simulink model "mrsMultiRobotAvoidance"  (R2024a)
settings: Solver=FixedStepAuto  StartTime=0.0  StopTime=inf  FixedStep=sampleTime  RelTol=1e-3
PreLoadFcn:
  | % Simulation parameters
  | load exampleMap
  | sampleTime = 0.05;
  | 
  | % Robot parameters
  | wheelRadius = 0.025;
  | robotRadius = 0.35;
  | 
  | % Lidar parameters
  | sensorOffset = [0,0];
  | scanAngles = linspace(-pi/2,pi/2,9)';
  | maxRange = 5;
undefined symbols (not defined in the file): detect_array, objDetectorAngle, objDetectorFOV, objDetectorOffset, objDetectorRange
libraries: mobileRoboticsLib x10
settings Model: Creator=scastro  LastModifiedBy=niyu2
settings SolverCC: AlgebraicLoopSolver=TrustRegion
settings DataIOCC: ReturnWorkspaceOutputs=off
settings DebuggingCC: UnconnectedInputMsg=warning  UnconnectedOutputMsg=warning  UnconnectedLineMsg=warning  PregeneratedLibrarySubsystemCodeDiagnostic=none  ArithmeticOperatorsInVariantConditions=warning
settings ModelReferenceCC: EnableRefExpFcnMdlSchedulingChecks=on
settings SFSimCC: SimUseLocalCustomCode=off  CustomCodeUndefinedFunction=UseInterfaceOnly
settings RTWCC: RTWUseLocalCustomCode=off  GPUComputeCapability=3.5

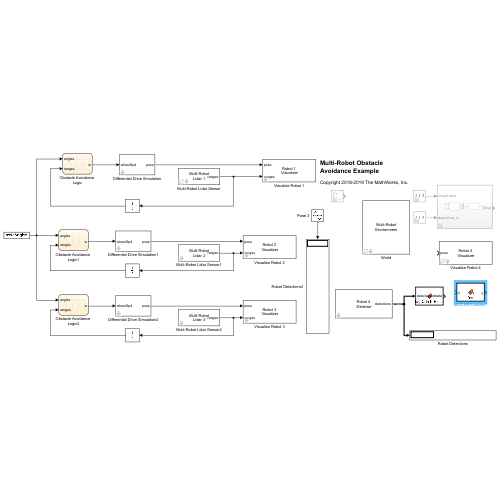
[thumbnail: Simulink's stored preview of the top-level diagram]
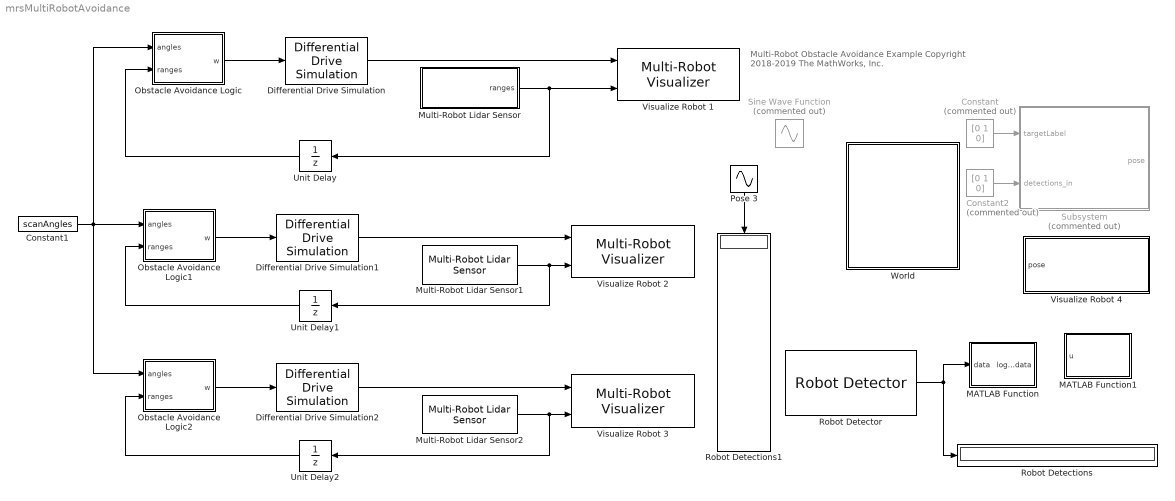
== system mrsMultiRobotAvoidance ==
  note: Multi-Robot Obstacle
      | Avoidance Example
      |
      | Copyright 2018-2019 The MathWorks, Inc.
  Constant : Constant  Commented=on  Value=[0 1 0]
  Constant1 : Constant  Value=scanAngles
  Constant2 : Constant  Commented=on  Value=[0 1 0]
  Differential Drive Simulation : mobileRoboticsLib/Kinematic Models/Differential Drive/Differential Drive Simulation  wheelRadius=wheelRadius  wheelBase=robotRadius  initX=4  initY=4  initAngle=0  Ts=sampleTime
      settings: SourceProductName=Mobile Robotics Simulation Toolbox
  Differential Drive Simulation1 : mobileRoboticsLib/Kinematic Models/Differential Drive/Differential Drive Simulation  wheelRadius=wheelRadius  wheelBase=robotRadius  initX=8  initY=8  initAngle=pi/2  Ts=sampleTime
      settings: SourceProductName=Mobile Robotics Simulation Toolbox
  Differential Drive Simulation2 : mobileRoboticsLib/Kinematic Models/Differential Drive/Differential Drive Simulation  wheelRadius=wheelRadius  wheelBase=robotRadius  initX=7.5  initY=3  initAngle=-pi/4  Ts=sampleTime
      settings: SourceProductName=Mobile Robotics Simulation Toolbox
  MATLAB Function : MATLAB Function  TreatAsAtomicUnit=on
  MATLAB Function1 : MATLAB Function  TreatAsAtomicUnit=on
  Multi-Robot Lidar Sensor : Subsystem  AncestorBlock=mobileRoboticsLib/Environments/Multi-Robot Lidar Sensor  mask(Multi-Robot Lidar Sensor){robotIdx=1, mapName=map, sensorOffset=sensorOffset, scanAngles=scanAngles, maxRange=maxRange}
      mask prompts: robotIdx "Robot Index"; mapName "Map Name"; sensorOffset "Sensor offset (x,y) [m]"; scanAngles "Scan angles [rad]"; maxRange "Maximum Range [m]"
      mask help: 2D lidar sensor simulation for multi-robot environment.
      mask init:
      | % Find number of robots 
      | mrEnvBlks = find_system(bdroot,'FollowLinks','on','LookUnderMasks','on','MaskType','Multi-Robot Environment');
      | mrEnvBlk = mrEnvBlks{1};
      | if isempty(mrEnvBlk)
      |     error('No Multi-Robot Environment found in model.')
      | end
      | numRobots = evalin('base',get_param(mrEnvBlk,'numRobots'));
      | 
      | % Configure pose tags
      | poseSub = [gcb '/Poses'];
      | poseBlocks = find_system(poseSub,'FollowLinks','on','LookUnderMasks','on','BlockType','From');
      | for idx = 1:numel(poseBlocks)
      |     lh = get_param(poseBlocks{idx},'LineHandles');
      |     delete_line(lh.Outport);
      | end
      | delete_block(poseBlocks);
      | vecBlock = [poseSub '/Vector Concatenate'];
      | set_param(vecBlock,'NumInputs',num2str(numRobots));
      | for idx = 1:numRobots
      |     blkName = [poseSub '/From' num2str(idx)];
      |     blkPos = [0 30 200 50] + (idx-1)*[0 30 0 30];
      |     add_block('simulink/Signal Routing/From',blkName);
      |     set_param(blkName,'GotoTag',['slMultiRobotEnv_Pose_' num2str(idx)]);
      |     set_param(blkName,'Position',blkPos);
      |     add_line(poseSub,['From' num2str(idx) '/1'],['Vector Concatenate/' num2str(idx)]);
      | end
      | 
      | % Configure visual tags
      | visualSub = [gcb '/Visuals'];
      | visualBlocks = find_system(visualSub,'FollowLinks','on','LookUnderMasks','on','BlockType','From');
      | for idx = 1:numel(visualBlocks)
      |     lh = get_param(visualBlocks{idx},'LineHandles');
      |     delete_line(lh.Outport);
      | end
      | delete_block(visualBlocks);
      | vecBlock = [visualSub '/Vector Concatenate'];
      | set_param(vecBlock,'NumInputs',num2str(numRobots));
      | for idx = 1:numRobots
      |     blkName = [visualSub '/From' num2str(idx)];
      |     blkPos = [0 30 200 50] + (idx-1)*[0 30 0 30];
      |     add_block('simulink/Signal Routing/From',blkName);
      |     set_param(blkName,'GotoTag',['slMultiRobotEnv_Visuals_' num2str(idx)]);
      |     set_param(blkName,'Position',blkPos);
      |     add_line(visualSub,['From' num2str(idx) '/1'],['Vector Concatenate/' num2str(idx)]);
      | end
      mask Help: web('matlab: edit mrsDocLidarSensor')
      mask Callback mapName:
      | % Update the map in the Robot Detector system object inside the mask
      | mapName = get_param(gcb,'mapName');
      | blkName = [gcb '/Multi-Robot Lidar Sensor'];
      | set_param(blkName,'mapName',mapName);
      mask Display:
      | idx = get_param(gcb,'robotIdx');
      | fprintf(['Multi Robot\nLidar ' idx])
  Multi-Robot Lidar Sensor1 : mobileRoboticsLib/Environments/Multi-Robot Lidar Sensor  robotIdx=2  mapName=map  sensorOffset=sensorOffset  scanAngles=scanAngles  maxRange=maxRange
      settings: SourceProductName=Mobile Robotics Simulation Toolbox
  Multi-Robot Lidar Sensor2 : mobileRoboticsLib/Environments/Multi-Robot Lidar Sensor  robotIdx=3  mapName=map  sensorOffset=sensorOffset  scanAngles=scanAngles  maxRange=maxRange
      settings: SourceProductName=Mobile Robotics Simulation Toolbox
  Obstacle Avoidance Logic : Stateflow chart  TreatAsAtomicUnit=on
  Obstacle Avoidance Logic1 : Stateflow chart  TreatAsAtomicUnit=on
  Obstacle Avoidance Logic2 : Stateflow chart  TreatAsAtomicUnit=on
  Pose 3 : Sin  SineType=Sample based  Amplitude=[-2;0.5;pi/2]  Bias=[7.75;3;0]  Phase=[-pi/4;0;pi/3]  Samples=160  SampleTime=sampleTime  Offset=[0;50;25]
  Robot Detections : Display
  Robot Detections1 : Display
  Robot Detector : mobileRoboticsLib/Environments/Robot Detector  mapName=map  robotIdx=4  sensorOffset=[0,0]  sensorAngle=0  sensorFOV=pi/3  maxRange=10  maxDetections=1  sampleTime=-1
      settings: SourceProductName=Mobile Robotics Simulation Toolbox
  Sine Wave Function : Sin  Commented=on  SineType=Sample based  Amplitude=[detect_array(1);detect_array(2);detect_array(3)]  Bias=[7.75;3;0]  Samples=160  SampleTime=0.05  Offset=[0;50;25]
  Subsystem : Subsystem  Commented=on
  Unit Delay : UnitDelay  SampleTime=-1  HasFrameUpgradeWarning=on
  Unit Delay1 : UnitDelay  SampleTime=-1  HasFrameUpgradeWarning=on
  Unit Delay2 : UnitDelay  SampleTime=-1  HasFrameUpgradeWarning=on
  Visualize Robot 1 : mobileRoboticsLib/Environments/Multi-Robot Visualizer  idx=1  radius=robotRadius  robotColor=[0 1 0]  showTraj=off  hasLidar=on  sensorOffset=sensorOffset  scanAngles=scanAngles  maxNumScans=0  hasObjDetector=off  objDetectorOffset=[0,0]  objDetectorAngle=0  objDetectorFOV=pi/2  objDetectorMaxRange=5  hasRobotDetector=off  robotDetectorOffset=[0,0]  robotDetectorAngle=0  robotDetectorFOV=pi/3  robotDetectorMaxRange=5  robotDetectorNumDetections=0
      settings: SourceProductName=Mobile Robotics Simulation Toolbox
  Visualize Robot 2 : mobileRoboticsLib/Environments/Multi-Robot Visualizer  idx=2  radius=robotRadius  robotColor=[0 0 1]  showTraj=on  hasLidar=on  sensorOffset=sensorOffset  scanAngles=scanAngles  maxNumScans=0  hasObjDetector=off  objDetectorOffset=[0 0]  objDetectorAngle=0  objDetectorFOV=pi/2  objDetectorMaxRange=5  hasRobotDetector=off  robotDetectorOffset=[0,0]  robotDetectorAngle=0  robotDetectorFOV=pi/3  robotDetectorMaxRange=5  robotDetectorNumDetections=0
      settings: SourceProductName=Mobile Robotics Simulation Toolbox
  Visualize Robot 3 : mobileRoboticsLib/Environments/Multi-Robot Visualizer  idx=3  radius=robotRadius  robotColor=[0 0 1]  showTraj=off  hasLidar=on  sensorOffset=sensorOffset  scanAngles=scanAngles  maxNumScans=0  hasObjDetector=off  objDetectorOffset=[0 0]  objDetectorAngle=0  objDetectorFOV=pi/2  objDetectorMaxRange=5  hasRobotDetector=off  robotDetectorOffset=[0,0]  robotDetectorAngle=0  robotDetectorFOV=pi/3  robotDetectorMaxRange=5  robotDetectorNumDetections=0
      settings: SourceProductName=Mobile Robotics Simulation Toolbox
  Visualize Robot 4 : Subsystem  AncestorBlock=mobileRoboticsLib/Environments/Multi-Robot Visualizer  mask(Multi-Robot Visualizer){idx=4, radius=0.25, robotColor=[0 0 1], showTraj=on, hasLidar=off, sensorOffset=sensorOffset, scanAngles=scanAngles, maxNumScans=0, hasObjDetector=off, objDetectorOffset=objDetectorOffset, objDetectorAngle=objDetectorAngle, objDetectorFOV=objDetectorFOV, objDetectorMaxRange=objDetectorRange, hasRobotDetector=on, robotDetectorOffset=[0,0], robotDetectorAngle=0, robotDetectorFOV=pi/3, robotDetectorMaxRange=10, robotDetectorNumDetections=0}
      mask prompts: idx "Robot Index"; radius "Robot Radius [m]"; robotColor "Robot Color"; showTraj "Show Trajectory"; hasLidar "Accept Lidar"; sensorOffset "Lidar sensor offset (x,y) [m]"; scanAngles "Scan angles [rad]"; maxNumScans "Maximum number of scans"; hasObjDetector "Accept Object Detector"; objDetectorOffset "Object detector offset (x,y) [m]"; objDetectorAngle "Object detector angle [rad]"; objDetectorFOV "Object detector field of view [rad]"; objDetectorMaxRange "Object detector maximum range [m]"; hasRobotDetector "Accept Robot Detector"; robotDetectorOffset "Robot detector offset (x,y) [m]"; robotDetectorAngle "Robot detector angle [rad]"; robotDetectorFOV "Robot detector field of view [rad]"; robotDetectorMaxRange "Robot detector maximum range [m]"; robotDetectorNumDetections "Maximum number of detections"
      mask help:
      | Supply the pose and (optionally) lidar ranges for a single robot in a multi-robot setup.
      |
      | These blocks require a "Multi-Robot Environment" block to exist in the model.
      mask init:
      | % Configure ranges port
      | if ~hasLidar & ~isempty(find_system(gcb,'FollowLinks','on','LookUnderMasks','on','BlockType','Inport','Name','ranges'))
      |     replace_block(gcb,'FollowLinks','on','Name','ranges','built-in/Ground','noprompt');
      | elseif hasLidar & isempty(find_system(gcb,'FollowLinks','on','LookUnderMasks','on','BlockType','Inport','Name','ranges'))
      |     replace_block(gcb,'FollowLinks','on','Name','ranges','built-in/Inport','noprompt');  
      | end
      | 
      | % Set up the Goto tag numbers
      | set_param([gcb '/Goto_Visuals'],'GotoTag',['slMultiRobotEnv_Visuals_' num2str(idx)]);
      | set_param([gcb '/Goto_Pose'],'GotoTag',['slMultiRobotEnv_Pose_' num2str(idx)]);
      | set_param([gcb '/Goto_Ranges'],'GotoTag',['slMultiRobotEnv_Ranges_' num2str(idx)]);
      | set_param([gcb '/Goto_ObjDetector'],'GotoTag',['slMultiRobotEnv_ObjDet_' num2str(idx)]);
      | set_param([gcb '/Goto_RobotDetector'],'GotoTag',['slMultiRobotEnv_RobotDet_' num2str(idx)]);
      | 
      | % Get the maximum number of scans
      | maxNumScans = internal.getMaxNumScans;
      | 
      | % Initialize range sensor bus
      | internal.createRangeSensorBus;
      mask Help: web('matlab: edit mrsDocMultiRobotEnv')
      mask Callback hasLidar:
      | mask = Simulink.Mask.get(gcb);
      | hasLidar = get_param(gcb,'hasLidar');
      | 
      | % Enable and disable parameters
      | indices = [find(strcmp({mask.Parameters.Name},'sensorOffset'));
      |            find(strcmp({mask.Parameters.Name},'scanAngles'))];
      | 
      | for idx = 1:numel(indices)
      |     mask.Parameters(indices(idx)).Visible = hasLidar;
      | end
      mask Callback hasObjDetector:
      | mask = Simulink.Mask.get(gcb);
      | hasObjDetector = get_param(gcb,'hasObjDetector');
      | 
      | indices = [find(strcmp({mask.Parameters.Name},'objDetectorOffset'));
      |            find(strcmp({mask.Parameters.Name},'objDetectorAngle'));
      |            find(strcmp({mask.Parameters.Name},'objDetectorFOV'));
      |            find(strcmp({mask.Parameters.Name},'objDetectorMaxRange'))];
      | 
      | for idx = 1:numel(indices)
      |     mask.Parameters(indices(idx)).Visible = hasObjDetector;
      | end
      mask Callback hasRobotDetector:
      | mask = Simulink.Mask.get(gcb);
      | hasObjDetector = get_param(gcb,'hasRobotDetector');
      | 
      | indices = [find(strcmp({mask.Parameters.Name},'robotDetectorOffset'));
      |            find(strcmp({mask.Parameters.Name},'robotDetectorAngle'));
      |            find(strcmp({mask.Parameters.Name},'robotDetectorFOV'));
      |            find(strcmp({mask.Parameters.Name},'robotDetectorMaxRange'))];
      | 
      | for idx = 1:numel(indices)
      |     mask.Parameters(indices(idx)).Visible = hasObjDetector;
      | end
      mask DialogControl Container4 Prompt: Robot
      mask DialogControl Container6 Prompt: Sensors
      mask Display:
      | idx = get_param(gcb,'idx');
      | fprintf(['Robot ' idx '\n Visualizer'])
  World : Subsystem  AncestorBlock=mobileRoboticsLib/Environments/Multi-Robot Environment  InitFcn=clear multiRobotVizWorld;  mask(Multi-Robot Environment){numRobots=4, mapName=map, showWaypoints=off, showObjects=off, objectColors=[1 0 0;0 1 0;0 0 1], objectMarkers='s', showRobotIds=on, plotSensorLines=on}
      mask prompts: numRobots "Number of Robots"; mapName "Map Name"; showWaypoints "Accept Waypoints"; showObjects "Accept Objects"; objectColors "Object Colors"; objectMarkers "Object Markers"; showRobotIds "Show Robot IDs"; plotSensorLines "Plot Sensor Lines"
      mask help:
      | Displays map, waypoint, and object data for a multi-robot simulation.
      |
      | Use "Multi-Robot Visualizer" blocks to display individual robots in this environment.
      mask init:
      | % Configure visual tags
      | visualSub = [gcb '/Visuals'];
      | radiusBlocks = find_system(visualSub,'FollowLinks','on','LookUnderMasks','on','BlockType','From');
      | for idx = 1:numel(radiusBlocks)
      |     lh = get_param(radiusBlocks{idx},'LineHandles');
      |     delete_line(lh.Outport);
      | end
      | delete_block(radiusBlocks);
      | vecBlock = [visualSub '/Vector Concatenate'];
      | set_param(vecBlock,'NumInputs',num2str(numRobots));
      | for idx = 1:numRobots
      |     blkName = [visualSub '/From' num2str(idx)];
      |     blkPos = [0 30 200 50] + (idx-1)*[0 30 0 30];
      |     add_block('simulink/Signal Routing/From',blkName);
      |     set_param(blkName,'GotoTag',['slMultiRobotEnv_Visuals_' num2str(idx)]);
      |     set_param(blkName,'Position',blkPos);
      |     add_line(visualSub,['From' num2str(idx) '/1'],['Vector Concatenate/' num2str(idx)]);
      | end
      | 
      | % Configure pose tags
      | poseSub = [gcb '/Poses'];
      | poseBlocks = find_system(poseSub,'FollowLinks','on','LookUnderMasks','on','BlockType','From');
      | for idx = 1:numel(poseBlocks)
      |     lh = get_param(poseBlocks{idx},'LineHandles');
      |     delete_line(lh.Outport);
      | end
      | delete_block(poseBlocks);
      | vecBlock = [poseSub '/Vector Concatenate'];
      | set_param(vecBlock,'NumInputs',num2str(numRobots));
      | for idx = 1:numRobots
      |     blkName = [poseSub '/From' num2str(idx)];
      |     blkPos = [0 30 200 50] + (idx-1)*[0 30 0 30];
      |     add_block('simulink/Signal Routing/From',blkName);
      |     set_param(blkName,'GotoTag',['slMultiRobotEnv_Pose_' num2str(idx)]);
      |     set_param(blkName,'Position',blkPos);
      |     add_line(poseSub,['From' num2str(idx) '/1'],['Vector Concatenate/' num2str(idx)]);
      | end
      | 
      | % Configure range tags
      | rangeSub = [gcb '/Ranges'];
      | rangeBlocks = find_system(rangeSub,'FollowLinks','on','LookUnderMasks','on','BlockType','From');
      | for idx = 1:numel(rangeBlocks)
      |     lh = get_param(rangeBlocks{idx},'LineHandles');
      |     delete_line(lh.Outport);
      | end
      | delete_block(rangeBlocks);
      | vecBlock = [rangeSub '/Vector Concatenate'];
      | set_param(vecBlock,'NumInputs',num2str(numRobots));
      | for idx = 1:numRobots
      |     blkName = [rangeSub '/From' num2str(idx)];
      |     blkPos = [0 30 200 50] + (idx-1)*[0 30 0 30];
      |     add_block('simulink/Signal Routing/From',blkName);
      |     set_param(blkName,'GotoTag',['slMultiRobotEnv_Ranges_' num2str(idx)]);
      |     set_param(blkName,'Position',blkPos);
      |     add_line(rangeSub,['From' num2str(idx) '/1'],['Vector Concatenate/' num2str(idx)]);
      | end
      | 
      | % Initialize range sensor bus
      | internal.createRangeSensorBus;
      | 
      | % Configure object detector tags
      | objDetSub = [gcb '/ObjectDetectorParams'];
      | objDetBlocks = find_system(objDetSub,'FollowLinks','on','LookUnderMasks','on','BlockType','From');
      | for idx = 1:numel(objDetBlocks)
      |     lh = get_param(objDetBlocks{idx},'LineHandles');
      |     delete_line(lh.Outport);
      | end
      | delete_block(objDetBlocks);
      | vecBlock = [objDetSub '/Vector Concatenate'];
      | set_param(vecBlock,'NumInputs',num2str(numRobots));
      | for idx = 1:numRobots
      |     blkName = [objDetSub '/From' num2str(idx)];
      |     blkPos = [0 30 200 50] + (idx-1)*[0 30 0 30];
      |     add_block('simulink/Signal Routing/From',blkName);
      |     set_param(blkName,'GotoTag',['slMultiRobotEnv_ObjDet_' num2str(idx)]);
      |     set_param(blkName,'Position',blkPos);
      |     add_line(objDetSub,['From' num2str(idx) '/1'],['Vector Concatenate/' num2str(idx)]);
      | end
      | 
      | % Configure robot detector tags
      | robotDetSub = [gcb '/RobotDetectorParams'];
      | robotDetBlocks = find_system(robotDetSub,'FollowLinks','on','LookUnderMasks','on','BlockType','From');
      | for idx = 1:numel(robotDetBlocks)
      |     lh = get_param(robotDetBlocks{idx},'LineHandles');
      |     delete_line(lh.Outport);
      | end
      | delete_block(robotDetBlocks);
      | vecBlock = [robotDetSub '/Vector Concatenate'];
      | set_param(vecBlock,'NumInputs',num2str(numRobots));
      | for idx = 1:numRobots
      |     blkName = [robotDetSub '/From' num2str(idx)];
      |     blkPos = [0 30 200 50] + (idx-1)*[0 30 0 30];
      |     add_block('simulink/Signal Routing/From',blkName);
      |     set_param(blkName,'GotoTag',['slMultiRobotEnv_RobotDet_' num2str(idx)]);
      |     set_param(blkName,'Position',blkPos);
      |     add_line(robotDetSub,['From' num2str(idx) '/1'],['Vector Concatenate/' num2str(idx)]);
      | end
      | 
      | % Configure waypoints port
      | hasWaypointPort = ~isempty(find_system(gcb,'FollowLinks','on','LookUnderMasks','on','BlockType','Inport','Name','waypoints'));
      | if ~showWaypoints & hasWaypointPort
      |     replace_block(gcb,'FollowLinks','on','Name','waypoints','built-in/Ground','noprompt');
      | elseif showWaypoints & ~hasWaypointPort
      |     replace_block(gcb,'FollowLinks','on','Name','waypoints','built-in/Inport','noprompt'); 
      | end
      |  
      | % Configure objects port
      | hasObjectPort = ~isempty(find_system(gcb,'FollowLinks','on','LookUnderMasks','on','BlockType','Inport','Name','objects'));
      | if ~showObjects & hasObjectPort
      |     replace_block(gcb,'FollowLinks','on','Name','objects','built-in/Ground','noprompt');
      | elseif showObjects & ~hasObjectPort
      |     replace_block(gcb,'FollowLinks','on','Name','objects','built-in/Inport','noprompt');  
      | end
      | 
      | % Ensure the waypoints and objects ports are organized correctly
      | if strcmp(get_param([gcb '/waypoints'],'BlockType'),'Inport')
      |     set_param([gcb '/waypoints'],'Port','1');
      | end
      mask Help: web('matlab: edit mrsDocMultiRobotEnv')
      mask Callback showObjects:
      | mask = Simulink.Mask.get(gcb);
      | showObjects = get_param(gcb,'showObjects');
      | 
      | % Enable and disable parameters
      | indices = [find(strcmp({mask.Parameters.Name},'objectColors'));
      |            find(strcmp({mask.Parameters.Name},'objectMarkers'))];
      | 
      | for idx = 1:numel(indices)
      |     mask.Parameters(indices(idx)).Visible = showObjects;
      | end
      mask Display: fprintf('Multi-Robot\nEnvironment')
  wires:
  Differential Drive Simulation/1 -> Visualize Robot 1/1
  Differential Drive Simulation1/1 -> Visualize Robot 2/1
  Obstacle Avoidance Logic/1(w) -> Differential Drive Simulation/1
  Unit Delay/1 -> Obstacle Avoidance Logic/2(ranges)
  Obstacle Avoidance Logic1/1(w) -> Differential Drive Simulation1/1
  Unit Delay1/1 -> Obstacle Avoidance Logic1/2(ranges)
  Unit Delay2/1 -> Obstacle Avoidance Logic2/2(ranges)
  Constant1/1 -> Obstacle Avoidance Logic2/1(angles), Obstacle Avoidance Logic1/1(angles), Obstacle Avoidance Logic/1(angles)
  Multi-Robot Lidar Sensor2/1 -> Visualize Robot 3/2, Unit Delay2/1
  Obstacle Avoidance Logic2/1(w) -> Differential Drive Simulation2/1
  Differential Drive Simulation2/1 -> Visualize Robot 3/1
  Multi-Robot Lidar Sensor/1(ranges) -> Unit Delay/1, Visualize Robot 1/2
  Multi-Robot Lidar Sensor1/1 -> Unit Delay1/1, Visualize Robot 2/2
  Pose 3/1 -> Robot Detections1/1
  Constant/1 -> Subsystem/1(targetLabel)
  Constant2/1 -> Subsystem/2(detections_in)
  Robot Detector/1 -> MATLAB Function/1(data), Robot Detections/1

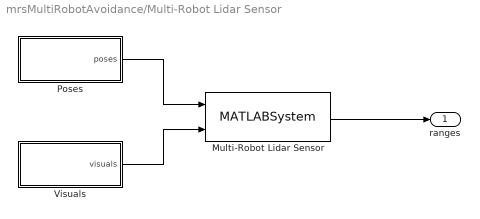
== system mrsMultiRobotAvoidance/Multi-Robot Lidar Sensor ==
  Multi-Robot Lidar Sensor : MATLABSystem  System=MultiRobotLidarSensor  mapName=map  sensorOffset=sensorOffset  scanAngles=scanAngles  maxRange=maxRange  robotIdx=robotIdx  robotRadii=-1
      mask Type: MultiRobotLidarSensor
      mask Display:
      | disp(['Multi-Robot' char(10) 'Lidar 1']);
      | port_label('output',1,'ranges');
  Poses : Subsystem
  Visuals : Subsystem
  ranges : Outport  VectorParamsAs1DForOutWhenUnconnected=off
  wires:
  Visuals/1(visuals) -> Multi-Robot Lidar Sensor/2
  Multi-Robot Lidar Sensor/1 -> ranges/1
  Poses/1(poses) -> Multi-Robot Lidar Sensor/1

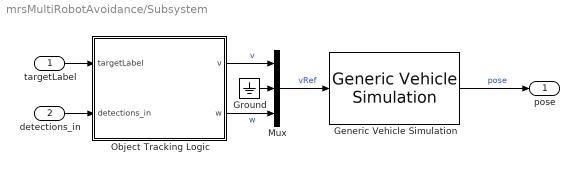
== system mrsMultiRobotAvoidance/Subsystem ==
  targetLabel : Inport
  detections_in : Inport  Port=2
  Generic Vehicle Simulation : mobileRoboticsLib/Utilities/Generic Vehicle Simulation  initX=2  initY=3  initAngle=0  Ts=sampleTime
      settings: SourceProductName=Mobile Robotics Simulation Toolbox
  Ground : Ground
  Mux : Mux  Inputs=3
  Object Tracking Logic : Stateflow chart  TreatAsAtomicUnit=on
  pose : Outport
  wires:
  targetLabel/1 -> Object Tracking Logic/1(targetLabel)
  Mux/1 -> Generic Vehicle Simulation/1  "vRef"
  Object Tracking Logic/2(w) -> Mux/3  "w"
  Object Tracking Logic/1(v) -> Mux/1  "v"
  detections_in/1 -> Object Tracking Logic/2(detections_in)
  Ground/1 -> Mux/2
  Generic Vehicle Simulation/1 -> pose/1  "pose"

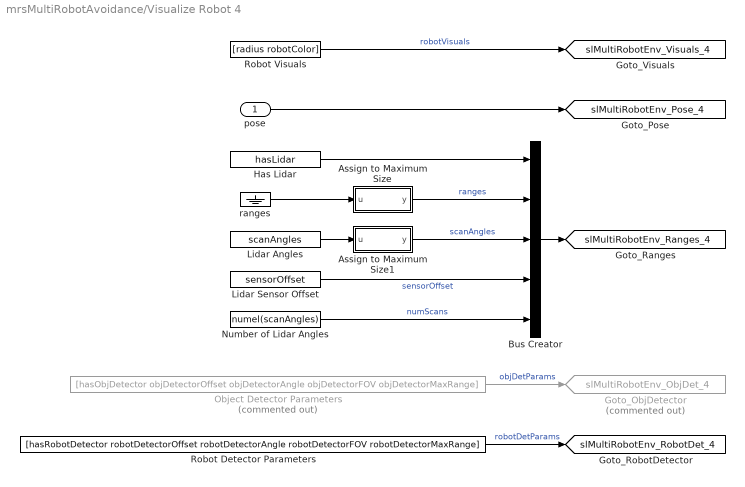
== system mrsMultiRobotAvoidance/Visualize Robot 4 ==
  pose : Inport
  Assign to Maximum Size : MATLAB Function  TreatAsAtomicUnit=on  mask{maxLength=maxNumScans}
      mask prompts: maxLength "Maximum Length"
  Assign to Maximum Size1 : MATLAB Function  TreatAsAtomicUnit=on  mask{maxLength=maxNumScans}
      mask prompts: maxLength "Maximum Length"
  Bus Creator : BusCreator  Inputs=5  OutDataTypeStr=Bus: slbus_MultiRobotRangeSensor  NonVirtualBus=on
      settings: InheritFromInputs=off
  Goto_ObjDetector : Goto  Commented=on  GotoTag=slMultiRobotEnv_ObjDet_4  TagVisibility=global
  Has Lidar : Constant  Value=hasLidar  OutDataTypeStr=boolean
  Lidar Angles : Constant  Value=scanAngles
  Lidar Sensor Offset : Constant  Value=sensorOffset
  Number of Lidar Angles : Constant  Value=numel(scanAngles)
  Object Detector Parameters : Constant  Commented=on  Value=[hasObjDetector objDetectorOffset objDetectorAngle objDetectorFOV objDetectorMaxRange]
  Robot Detector Parameters : Constant  Value=[hasRobotDetector robotDetectorOffset robotDetectorAngle robotDetectorFOV robotDetectorMaxRange]
  Robot Visuals : Constant  Value=[radius robotColor]
  ranges : Ground
  tag scope: slMultiRobotEnv_Pose_4=global, slMultiRobotEnv_Ranges_4=global, slMultiRobotEnv_RobotDet_4=global, slMultiRobotEnv_Visuals_4=global
  wires:
  Has Lidar/1 -> Bus Creator/1
  Robot Detector Parameters/1 -> [slMultiRobotEnv_RobotDet_4]  "robotDetParams"
  Object Detector Parameters/1 -> Goto_ObjDetector/1  "objDetParams"
  Robot Visuals/1 -> [slMultiRobotEnv_Visuals_4]  "robotVisuals"
  Number of Lidar Angles/1 -> Bus Creator/5  "numScans"
  Assign to Maximum Size1/1(y) -> Bus Creator/3  "scanAngles"
  Lidar Angles/1 -> Assign to Maximum Size1/1(u)
  Assign to Maximum Size/1(y) -> Bus Creator/2  "ranges"
  Lidar Sensor Offset/1 -> Bus Creator/4  "sensorOffset"
  Bus Creator/1 -> [slMultiRobotEnv_Ranges_4]
  ranges/1 -> Assign to Maximum Size/1(u)
  pose/1 -> [slMultiRobotEnv_Pose_4]

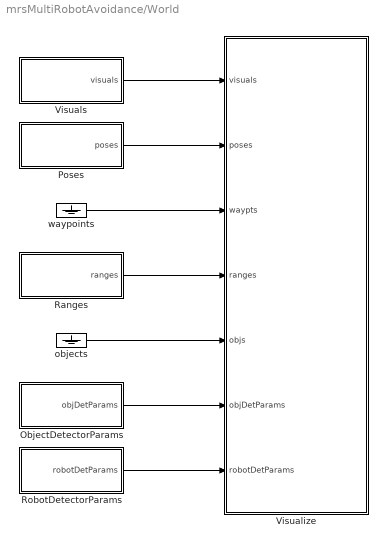
== system mrsMultiRobotAvoidance/World ==
  ObjectDetectorParams : Subsystem
  Poses : Subsystem
  Ranges : Subsystem
  RobotDetectorParams : Subsystem
  Visualize : MATLAB Function  TreatAsAtomicUnit=on
  Visuals : Subsystem
  objects : Ground
  waypoints : Ground
  wires:
  objects/1 -> Visualize/5(objs)
  waypoints/1 -> Visualize/3(waypts)
  Ranges/1(ranges) -> Visualize/4(ranges)
  Poses/1(poses) -> Visualize/2(poses)
  Visuals/1(visuals) -> Visualize/1(visuals)
  ObjectDetectorParams/1(objDetParams) -> Visualize/6(objDetParams)
  RobotDetectorParams/1(robotDetParams) -> Visualize/7(robotDetParams)

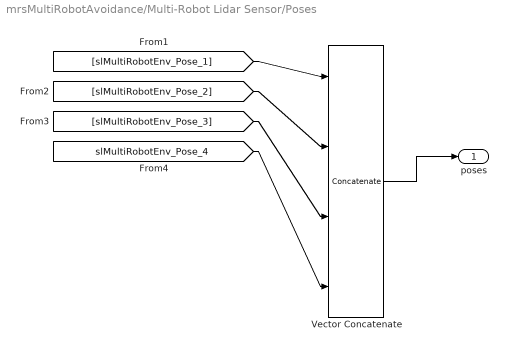
== system mrsMultiRobotAvoidance/Multi-Robot Lidar Sensor/Poses ==
  Vector Concatenate : Concatenate  NumInputs=4  Mode=Multidimensional array  ConcatenateDimension=2
  poses : Outport
  wires:
  Vector Concatenate/1 -> poses/1
  [slMultiRobotEnv_Pose_1] -> Vector Concatenate/1
  [slMultiRobotEnv_Pose_2] -> Vector Concatenate/2
  [slMultiRobotEnv_Pose_3] -> Vector Concatenate/3
  [slMultiRobotEnv_Pose_4] -> Vector Concatenate/4

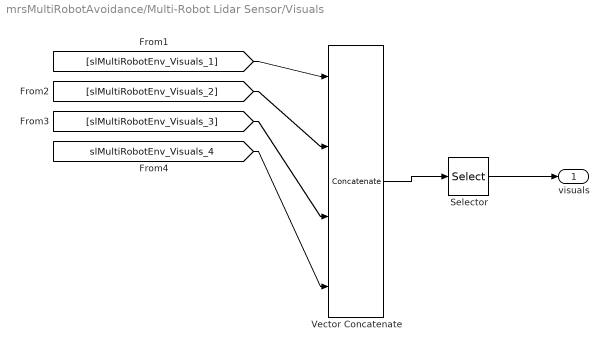
== system mrsMultiRobotAvoidance/Multi-Robot Lidar Sensor/Visuals ==
  Selector : Selector  NumberOfDimensions=2  InputPortWidth=3  IndexOptions=Index vector (dialog),Select all  Indices=1,1  OutputSizes=1,1
  Vector Concatenate : Concatenate  NumInputs=4  Mode=Multidimensional array  ConcatenateDimension=2
  visuals : Outport
  wires:
  Selector/1 -> visuals/1
  Vector Concatenate/1 -> Selector/1
  [slMultiRobotEnv_Visuals_1] -> Vector Concatenate/1
  [slMultiRobotEnv_Visuals_2] -> Vector Concatenate/2
  [slMultiRobotEnv_Visuals_3] -> Vector Concatenate/3
  [slMultiRobotEnv_Visuals_4] -> Vector Concatenate/4

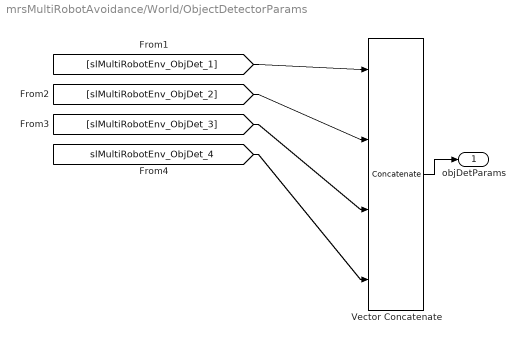
== system mrsMultiRobotAvoidance/World/ObjectDetectorParams ==
  Vector Concatenate : Concatenate  NumInputs=4  Mode=Multidimensional array  ConcatenateDimension=2
  objDetParams : Outport
  wires:
  Vector Concatenate/1 -> objDetParams/1
  [slMultiRobotEnv_ObjDet_1] -> Vector Concatenate/1
  [slMultiRobotEnv_ObjDet_2] -> Vector Concatenate/2
  [slMultiRobotEnv_ObjDet_3] -> Vector Concatenate/3
  [slMultiRobotEnv_ObjDet_4] -> Vector Concatenate/4

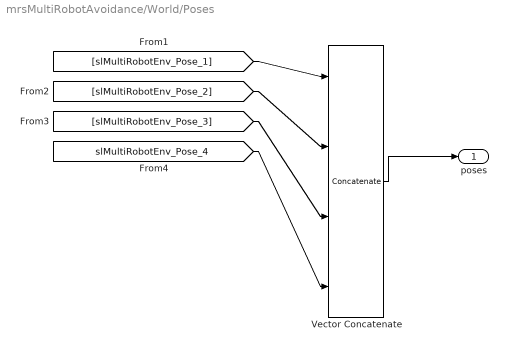
== system mrsMultiRobotAvoidance/World/Poses ==
  Vector Concatenate : Concatenate  NumInputs=4  Mode=Multidimensional array  ConcatenateDimension=2
  poses : Outport
  wires:
  Vector Concatenate/1 -> poses/1
  [slMultiRobotEnv_Pose_1] -> Vector Concatenate/1
  [slMultiRobotEnv_Pose_2] -> Vector Concatenate/2
  [slMultiRobotEnv_Pose_3] -> Vector Concatenate/3
  [slMultiRobotEnv_Pose_4] -> Vector Concatenate/4

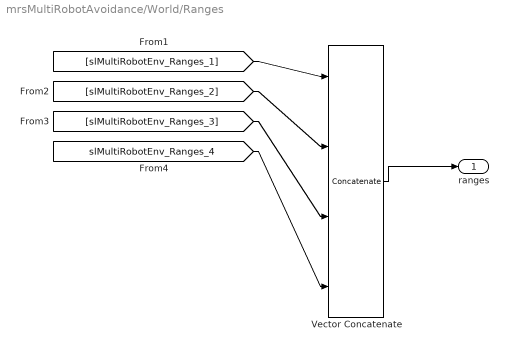
== system mrsMultiRobotAvoidance/World/Ranges ==
  Vector Concatenate : Concatenate  NumInputs=4  Mode=Multidimensional array  ConcatenateDimension=2
  ranges : Outport
  wires:
  Vector Concatenate/1 -> ranges/1
  [slMultiRobotEnv_Ranges_1] -> Vector Concatenate/1
  [slMultiRobotEnv_Ranges_2] -> Vector Concatenate/2
  [slMultiRobotEnv_Ranges_3] -> Vector Concatenate/3
  [slMultiRobotEnv_Ranges_4] -> Vector Concatenate/4

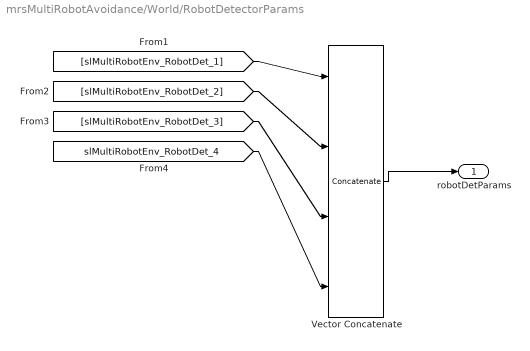
== system mrsMultiRobotAvoidance/World/RobotDetectorParams ==
  Vector Concatenate : Concatenate  NumInputs=4  Mode=Multidimensional array  ConcatenateDimension=2
  robotDetParams : Outport
  wires:
  Vector Concatenate/1 -> robotDetParams/1
  [slMultiRobotEnv_RobotDet_1] -> Vector Concatenate/1
  [slMultiRobotEnv_RobotDet_2] -> Vector Concatenate/2
  [slMultiRobotEnv_RobotDet_3] -> Vector Concatenate/3
  [slMultiRobotEnv_RobotDet_4] -> Vector Concatenate/4

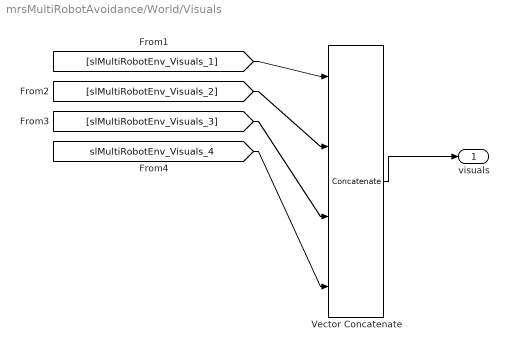
== system mrsMultiRobotAvoidance/World/Visuals ==
  Vector Concatenate : Concatenate  NumInputs=4  Mode=Multidimensional array  ConcatenateDimension=2
  visuals : Outport
  wires:
  Vector Concatenate/1 -> visuals/1
  [slMultiRobotEnv_Visuals_1] -> Vector Concatenate/1
  [slMultiRobotEnv_Visuals_2] -> Vector Concatenate/2
  [slMultiRobotEnv_Visuals_3] -> Vector Concatenate/3
  [slMultiRobotEnv_Visuals_4] -> Vector Concatenate/4

== stateflow chart mrsMultiRobotAvoidance/Obstacle Avoidance Logic2 ==
  state MainState [parallel]
    en,du:
    validIdx = ~isnan(ranges);
    validRanges = ranges(validIdx);
    validAngles = angles(validIdx);
    settings: executionOrder=1
    state Turn
      en,du:
      avgAngle = mean(validAngles./validRanges);
      state Left
        en, du:
        w = [0;12.5];
      state Right
        en, du:
        w = [12.5;0];
      (default) -> (junction 39)
      (junction 39) -> Left [order 1] : [avgAngle < 0]
      (junction 39) -> (junction 43) [order 2]
      Left -> Right : [after(1,sec) && ...
          | avgAngle > 0]
      Right -> Left : [after(1,sec) && ...
          | avgAngle < 0]
      (junction 43) -> Right
    state GoStraight
      en:
      w = [25; 25];
    (default) -> GoStraight
    GoStraight -> Turn : [any(validRanges<=1)]
    Turn -> GoStraight : [all(validRanges>1)]
  data: angles input; w output; ranges input; validRanges local size=numel(scanAngles); validIdx local; validAngles local size=numel(scanAngles); avgAngle local

== stateflow chart mrsMultiRobotAvoidance/Obstacle Avoidance Logic ==
  state MainState [parallel]
    en,du:
    validIdx = ~isnan(ranges);
    validRanges = ranges(validIdx);
    validAngles = angles(validIdx);
    settings: executionOrder=1
    state Turn
      en,du:
      avgAngle = mean(validAngles./validRanges);
      state Left
        en, du:
        w = [0;12.5];
      state Right
        en, du:
        w = [12.5;0];
      (default) -> (junction 39)
      (junction 39) -> Left [order 1] : [avgAngle < 0]
      (junction 39) -> (junction 43) [order 2]
      Left -> Right : [after(1,sec) && ...
          | avgAngle > 0]
      Right -> Left : [after(1,sec) && ...
          | avgAngle < 0]
      (junction 43) -> Right
    state GoStraight
      en:
      w = [25; 25];
    (default) -> GoStraight
    GoStraight -> Turn : [any(validRanges<=1)]
    Turn -> GoStraight : [all(validRanges>1)]
  data: angles input; w output; ranges input; validRanges local size=numel(scanAngles); validIdx local; validAngles local size=numel(scanAngles); avgAngle local

== matlab function mrsMultiRobotAvoidance/MATLAB Function ==
  data: data input; loggeddata output
function loggeddata = logDataToExcel(data)
% Appends variable-size data to an Excel file
persistent loggedData

% Initialize persistent variable on the first call
if isempty(loggedData)
    loggedData = {};
end

% Append current data
loggedData{end+1} = data;

% Save to Excel after simulation
assignin('base', 'loggedData', loggedData); % Save loggedData to base workspace
loggeddata = loggedData
end

== matlab function mrsMultiRobotAvoidance/MATLAB Function1 ==
  data: u input
function fcn(u)
% Assume the variable loggedData contains the data logged from Simulink

% Example loggedData structure:
% loggedData is a cell array where each cell contains a 3-element vector
% Each row represents a time step.

% Initialize a matrix or cell array for storing data
allData = [];

% Loop through each time step
for i = 1:length(u)
    % Extract the current data (assumed to be a 3-element vector)
    timeStepData = u{i}; % Access data for the time step (3-element vector)
    
    % Add the time step index (if needed)
    timeStep = i; % Current time step index
    
    % Append the time step and data as a new row
    allData = [allData; timeStep, timeStepData(:)']; % Ensure it's row format
end

% Convert the processed data to a table for easier Excel export
% Columns: TimeStep, Data1, Data2, Data3
outputTable = array2table(allData, 'VariableNames', {'TimeStep', 'Data1', 'Data2', 'Data3'});

% Save to Excel
filename = 'SimulinkOutput.xlsx';
writetable(outputTable, filename);

disp(['Data saved to ', filename]);

== stateflow chart mrsMultiRobotAvoidance/Subsystem/Object Tracking Logic ==
  state TrackObject
    entry, during:
    [range,angle,valid] = findValidObject(targetLabel);
    if valid
    count = 0;
    else
    count = count + 1;
    end
    (default) -> (junction 20)
    TrackObject -> (junction 20) [order 1]
    (junction 20) -> (junction 24) [order 1] : % Set angular speed if
        | % angle outside deadband
        | [abs(angle) > pi/24]
    (junction 20) -> (junction 30) [order 2] : {w = 0;}
    (junction 24) -> (junction 49) : % Proportional
        | % control
        | {w = 1.5*angle;}
    (junction 49) -> (junction 30)
    (junction 30) -> (junction 54)
    (junction 54) -> (junction 56) [order 1] : % Go forward if object is far
        | [range > 1]
    (junction 54) -> (junction 60) [order 2] : {v = 0;}
    (junction 56) -> (junction 58) : {v = 0.5;}
    (junction 58) -> (junction 60)
  state SeekObject
    entry:
    v = 0;
    w = 1;
  (default) -> TrackObject : {
      | count = 0;
      | range = 0;
      | angle = 0;
      | }
  TrackObject -> SeekObject [order 1] : [count > 20]
  SeekObject -> TrackObject : [~isempty(detections_in)]
  data: dist function_output; ang function_output; flag function_output; label function_input; targetLabel input; detections_in input fixdt(1,16,0) size=[objDetectorMaxHits,3]; v output; w output; angle local; range local; count local; valid local
  function [dist,ang,flag] = findValidObject(label):
    | function [dist,ang,flag] = findValidObject(label)
    | % Finds the distance (dist) and angle (ang) of the nearest valid
    | % object detected. If an object is found, the (flag) output is true.
    | 
    | % Initialize
    | flag = false;
    | dist = 0;
    | ang = 0;
    | 
    | if ~isempty(detections_in)
    |     % Loop through all detections
    |     for idx = 1:size(detections_in,1)
    |         % If a detection matching the target label is found, 
    |         % return it and set the valid flag to true.
    |         if detections_in(idx,3) == label
    |             dist = detections_in(idx,1);
    |             ang  = detections_in(idx,2);
    |             flag = true;
    |             return; 
    |         end
    |     end
    | end

== matlab function mrsMultiRobotAvoidance/World/Visualize ==
  data: visuals input; poses input; waypts input; numRobots parameter; ranges input; objs input; objDetParams input; robotDetParams input; plotSensorLines parameter; showRobotIds parameter
function visualizeWaypointsAndObjects(visuals,poses,waypts,numRobots,ranges,objs, ...
                                      objDetParams,robotDetParams,plotSensorLines, showRobotIds)

    coder.extrinsic('internal.multiRobotVizWorld')
    internal.multiRobotVizWorld(numRobots,visuals,poses,waypts,ranges,objs, ... 
                                objDetParams,robotDetParams,showRobotIds,plotSensorLines);

end

== matlab function mrsMultiRobotAvoidance/Visualize Robot 4/Assign to Maximum Size ==
  data: u input; y output size=maxLength; maxLength parameter
function y = assign2max(u,maxLength)

y = zeros(maxLength,1);
numElems = min(maxLength,size(u,1));
y(1:numElems) = u(1:numElems);

== matlab function mrsMultiRobotAvoidance/Visualize Robot 4/Assign to Maximum Size1 ==
  data: u input; y output size=maxLength; maxLength parameter
function y = assign2max(u,maxLength)

y = zeros(maxLength,1);
numElems = min(maxLength,size(u,1));
y(1:numElems) = u(1:numElems);

== stateflow chart mrsMultiRobotAvoidance/Obstacle Avoidance Logic1 ==
  state MainState [parallel]
    en,du:
    validIdx = ~isnan(ranges);
    validRanges = ranges(validIdx);
    validAngles = angles(validIdx);
    settings: executionOrder=1
    state Turn
      en,du:
      avgAngle = mean(validAngles./validRanges);
      state Left
        en, du:
        w = [0;12.5];
      state Right
        en, du:
        w = [12.5;0];
      (default) -> (junction 39)
      (junction 39) -> Left [order 1] : [avgAngle < 0]
      (junction 39) -> (junction 43) [order 2]
      Left -> Right : [after(1,sec) && ...
          | avgAngle > 0]
      Right -> Left : [after(1,sec) && ...
          | avgAngle < 0]
      (junction 43) -> Right
    state GoStraight
      en:
      w = [25; 25];
    (default) -> GoStraight
    GoStraight -> Turn : [any(validRanges<=1)]
    Turn -> GoStraight : [all(validRanges>1)]
  data: angles input; w output; ranges input; validRanges local size=numel(scanAngles); validIdx local; validAngles local size=numel(scanAngles); avgAngle local
